simulink model "OTHex_Mocap_data"  (R2015b)
settings: Solver=VariableStepAuto  StartTime=0.0  StopTime=Inf  RelTol=1e-3
undefined symbols (not defined in the file or in its folder): motion_capture_rate
libraries: genomix x4
settings Model: Creator=smishra  LastModifiedBy=smishra

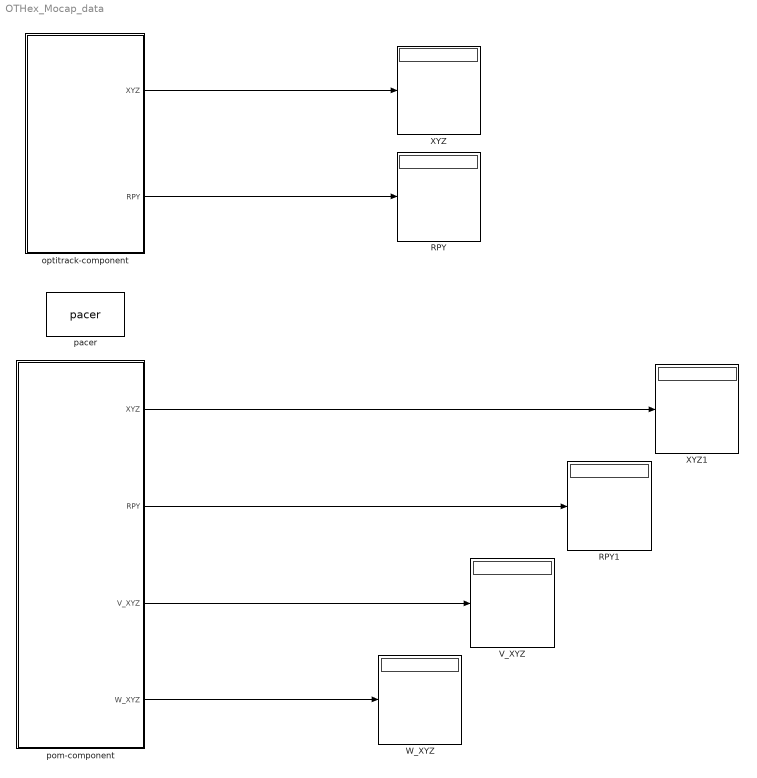
== system OTHex_Mocap_data ==
  RPY : Display
  RPY1 : Display
  V_XYZ : Display
  W_XYZ : Display
  XYZ : Display
  XYZ1 : Display
  optitrack-component : Subsystem
  pacer : genomix/pacer  Priority=0  catchup=off
  pom-component : Subsystem
  wires:
  optitrack-component/1(XYZ) -> XYZ/1
  optitrack-component/2(RPY) -> RPY/1
  pom-component/1(XYZ) -> XYZ1/1
  pom-component/2(RPY) -> RPY1/1
  pom-component/3(V_XYZ) -> V_XYZ/1
  pom-component/4(W_XYZ) -> W_XYZ/1

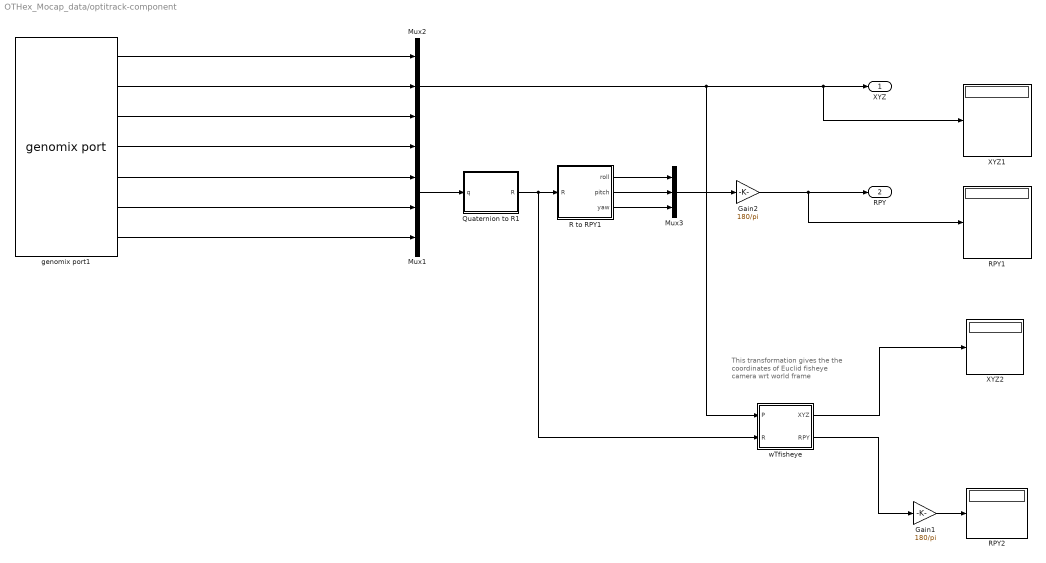
== system OTHex_Mocap_data/optitrack-component ==
  note: This transformation gives the
      | the coordinates of Euclid fisheye
      | camera wrt world frame
  Gain1 : Gain  Gain=180/pi
  Gain2 : Gain  Gain=180/pi
  Mux1 : Mux
  Mux2 : Mux  Inputs=3
  Mux3 : Mux  Inputs=3
  Quaternion to R1 : MATLAB Function  SystemSampleTime=motion_capture_rate
  R to RPY1 : MATLAB Function  TreatAsAtomicUnit=on
  RPY1 : Display
  RPY2 : Display
  XYZ1 : Display
  XYZ2 : Display
  genomix port1 : genomix/genomix port  host=localhost  component=optitrack  port=bodies  subport=OTHex  sigtype=value  timetype=periodic  period=0.01  siglist="[{\"name\":\"bodies.pos.x\",\"type\":\"value\",\"size\":1},{\"name\":\"bodies.pos.y\",\"type\":\"value\",\"size\":1},{\"name\":\"bodies.pos.z\",\"type\":\"value\",\"size\":1},{\"name\":\"bodies.pos.qw\",\"type\":\"value\",\"size\":1},{\"name\":\"bodies.pos.qx\",\"type\":\"value\",\"size\":1},{\"name\":\"bodies.pos.qy\",\"type\":\"value\",\"size\":1},{\"name\":\"bodies.pos.qz\",\"type\":\"value\",\"size\":1}]"
      settings: AttributesFormatString=optitrack/bodies
  wTfisheye : MATLAB Function  SystemSampleTime=motion_capture_rate
  XYZ : Outport
  RPY : Outport  Port=2
  wires:
  Mux3/1 -> Gain2/1
  R to RPY1/3(yaw) -> Mux3/3
  Gain2/1 -> RPY1/1, RPY/1
  genomix port1/3 -> Mux2/3
  genomix port1/6 -> Mux1/3
  R to RPY1/1(roll) -> Mux3/1
  R to RPY1/2(pitch) -> Mux3/2
  Mux2/1 -> wTfisheye/1(P), XYZ1/1, XYZ/1
  genomix port1/5 -> Mux1/2
  genomix port1/1 -> Mux2/1
  Mux1/1 -> Quaternion to R1/1(q)
  Quaternion to R1/1(R) -> wTfisheye/2(R), R to RPY1/1(R)
  genomix port1/2 -> Mux2/2
  genomix port1/7 -> Mux1/4
  genomix port1/4 -> Mux1/1
  wTfisheye/1(XYZ) -> XYZ2/1
  Gain1/1 -> RPY2/1
  wTfisheye/2(RPY) -> Gain1/1

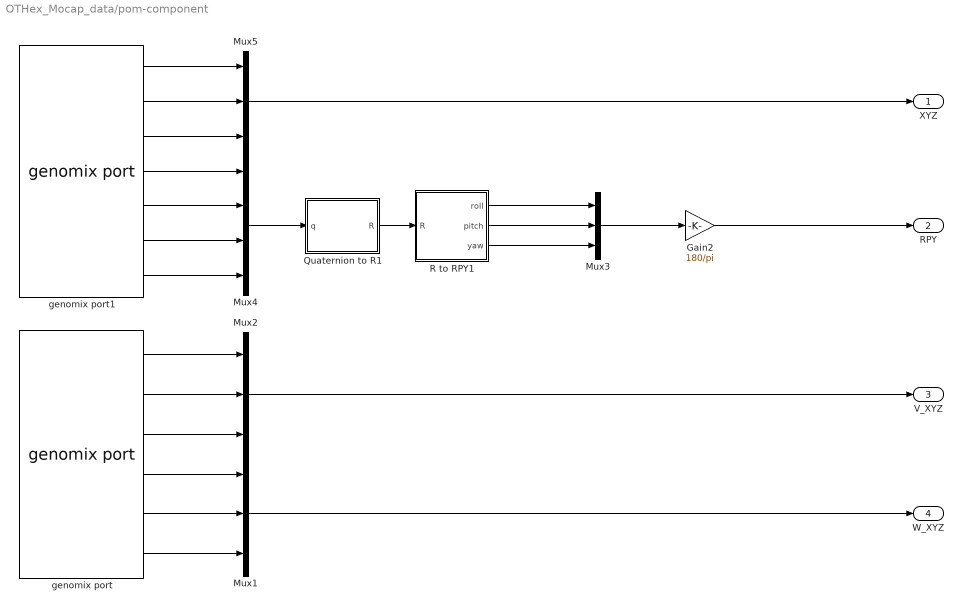
== system OTHex_Mocap_data/pom-component ==
  Gain2 : Gain  Gain=180/pi
  Mux{1..3,5} (4 alike) : Mux  Inputs=3
  Mux4 : Mux
  Quaternion to R1 : MATLAB Function  SystemSampleTime=motion_capture_rate
  R to RPY1 : MATLAB Function  TreatAsAtomicUnit=on
  genomix port : genomix/genomix port  host=localhost  component=pom  port=frame  subport=robot  sigtype=value  timetype=periodic  period=0.1  siglist="[{\"name\":\"frame.vel.vx\",\"type\":\"value\",\"size\":1},{\"name\":\"frame.vel.vy\",\"type\":\"value\",\"size\":1},{\"name\":\"frame.vel.vz\",\"type\":\"value\",\"size\":1},{\"name\":\"frame.vel.wx\",\"type\":\"value\",\"size\":1},{\"name\":\"frame.vel.wy\",\"type\":\"value\",\"size\":1},{\"name\":\"frame.vel.wz\",\"type\":\"value\",\"size\":1}]"
      settings: AttributesFormatString=pom/frame
  genomix port1 : genomix/genomix port  host=localhost  component=pom  port=frame  subport=robot  sigtype=value  timetype=periodic  period=0.1  siglist="[{\"name\":\"frame.pos.x\",\"type\":\"value\",\"size\":1},{\"name\":\"frame.pos.y\",\"type\":\"value\",\"size\":1},{\"name\":\"frame.pos.z\",\"type\":\"value\",\"size\":1},{\"name\":\"frame.pos.qw\",\"type\":\"value\",\"size\":1},{\"name\":\"frame.pos.qx\",\"type\":\"value\",\"size\":1},{\"name\":\"frame.pos.qy\",\"type\":\"value\",\"size\":1},{\"name\":\"frame.pos.qz\",\"type\":\"value\",\"size\":1}]"
      settings: AttributesFormatString=pom/frame
  XYZ : Outport
  RPY : Outport  Port=2
  V_XYZ : Outport  Port=3
  W_XYZ : Outport  Port=4
  wires:
  Mux2/1 -> V_XYZ/1
  genomix port/1 -> Mux2/1
  genomix port/4 -> Mux1/1
  genomix port/3 -> Mux2/3
  genomix port/5 -> Mux1/2
  Gain2/1 -> RPY/1
  genomix port/6 -> Mux1/3
  genomix port1/3 -> Mux5/3
  genomix port1/4 -> Mux4/1
  genomix port1/2 -> Mux5/2
  R to RPY1/1(roll) -> Mux3/1
  R to RPY1/2(pitch) -> Mux3/2
  Mux4/1 -> Quaternion to R1/1(q)
  Quaternion to R1/1(R) -> R to RPY1/1(R)
  Mux3/1 -> Gain2/1
  R to RPY1/3(yaw) -> Mux3/3
  genomix port1/1 -> Mux5/1
  Mux5/1 -> XYZ/1
  genomix port1/7 -> Mux4/4
  genomix port1/5 -> Mux4/2
  Mux1/1 -> W_XYZ/1
  genomix port1/6 -> Mux4/3
  genomix port/2 -> Mux2/2

== matlab function OTHex_Mocap_data/optitrack-component/Quaternion to R1 ==
  data: q input; R output
function R = fcn(q)

R=eye(3);

eta=q(1);
ex=q(2);
ey=q(3);
ez=q(4);

R=[2*(eta^2+ex^2)-1 2*(ex*ey-eta*ez) 2*(ex*ez+eta*ey);
2*(ex*ey+eta*ez) 2*(eta^2+ey^2)-1 2*(ey*ez-eta*ex);
2*(ex*ez-eta*ey) 2*(ey*ez+eta*ex) 2*(eta^2+ez^2)-1];

RCorrect=[1 0 0;0 -1 0; 0 0 -1];
% R=RCorrect*R;

== matlab function OTHex_Mocap_data/optitrack-component/R to RPY1 ==
  data: R input; roll output; pitch output; yaw output
function [roll,pitch,yaw] = fcn(R)

roll = atan2(R(3,2),R(3,3));
pitch = atan2(-R(3,1),sqrt(R(3,2)^2+R(3,3)^2));
yaw = atan2(R(2,1),R(1,1));

end

== matlab function OTHex_Mocap_data/pom-component/Quaternion to R1 ==
  data: q input; R output
function R = fcn(q)

R=eye(3);

eta=q(1);
ex=q(2);
ey=q(3);
ez=q(4);

R=[2*(eta^2+ex^2)-1 2*(ex*ey-eta*ez) 2*(ex*ez+eta*ey);
2*(ex*ey+eta*ez) 2*(eta^2+ey^2)-1 2*(ey*ez-eta*ex);
2*(ex*ez-eta*ey) 2*(ey*ez+eta*ex) 2*(eta^2+ez^2)-1];

RCorrect=[1 0 0;0 -1 0; 0 0 -1];
% R=RCorrect*R;

== matlab function OTHex_Mocap_data/pom-component/R to RPY1 ==
  data: R input; roll output; pitch output; yaw output
function [roll,pitch,yaw] = fcn(R)

roll = atan2(R(3,2),R(3,3));
pitch = atan2(-R(3,1),sqrt(R(3,2)^2+R(3,3)^2));
yaw = atan2(R(2,1),R(1,1));

end

== matlab function OTHex_Mocap_data/optitrack-component/wTfisheye ==
  data: P input; R input; XYZ output; RPY output
function [XYZ, RPY] = fcn(P,R)
% The following the displacement from the imu origin to the euclid's
% fisheye camera origin, measurements done with a simple ruler
% the rotation between the imu frame and the fisheye camera is identity
% x = 2.5 cm;
% y = 4.5 cm;
% z = 6.5 cm;

imuTfisheye = [eye(3,3) [0.025; 0.045; 0.065]
               0 0 0 1];
worldTimu = [R P; 0 0 0 1];

worldTfisheye = worldTimu * imuTfisheye;

XYZ = worldTfisheye(1:3,4);

worldRfisheye = worldTfisheye(1:3,1:3);
roll = atan2(worldRfisheye(3,2),worldRfisheye(3,3));
pitch = atan2(-worldRfisheye(3,1),sqrt(worldRfisheye(3,2)^2+worldRfisheye(3,3)^2));
yaw = atan2(worldRfisheye(2,1),worldRfisheye(1,1));

RPY = [roll; pitch; yaw];

end
